simulink model "DSB"  (R2022a)
settings: Solver=VariableStepAuto  StartTime=0.0  StopTime=9  RelTol=1e-3
InitFcn:
  | dsb_init()
StopFcn:
  | dsb_plots()
  | dsb_play()
libraries: commanapbnd3 x2, commchan3 x1
settings Model: Creator=aliel  LastModifiedBy=aliel

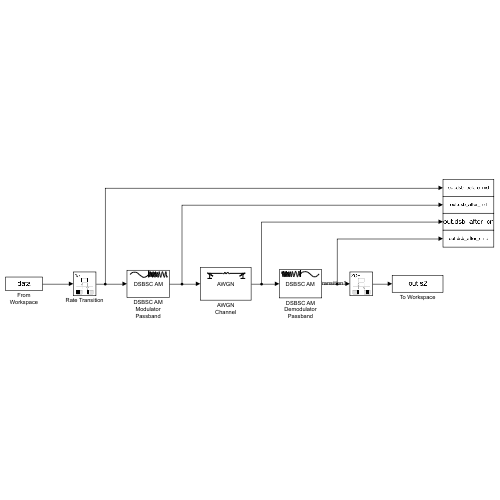
[thumbnail: Simulink's stored preview of the top-level diagram]
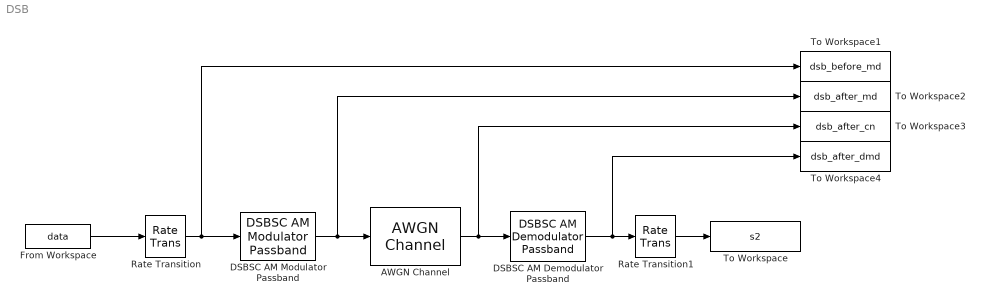
== system DSB ==
  AWGN Channel : commchan3/AWGN Channel  InputProcessing=Columns as channels (frame based)  seed=67  noiseMode="Signal to noise ratio  (SNR)"  EbNodB=10  EsNodB=10  SNRdB=30  bitsPerSym=1  Ps=0.0191  Tsym=1  variance=1
  DSBSC AM Demodulator Passband : commanapbnd3/DSBSC AM Demodulator Passband  Fc=17000  Ph=0  method=Chebyshev I  n=10  cf=4000  Rp=0.1  Rs=50
      settings: SourceProductBaseCode=CM
  DSBSC AM Modulator Passband : commanapbnd3/DSBSC AM Modulator Passband  Fc=17000  Ph=0
      settings: SourceProductBaseCode=CM
  From Workspace : FromWorkspace  VariableName=data  SampleTime=1/8192  OutputAfterFinalValue=Holding final value
  Rate Transition : RateTransition  OutPortSampleTime=1/(10*8192)
  Rate Transition1 : RateTransition  OutPortSampleTime=1/8192
  To Workspace : ToWorkspace  VariableName=s2  SampleTime=-1
      settings: Save2DSignal=2-D array (concatenate along first dimension)
  To Workspace1 : ToWorkspace  VariableName=dsb_before_md  SampleTime=-1
      settings: Save2DSignal=2-D array (concatenate along first dimension)
  To Workspace2 : ToWorkspace  VariableName=dsb_after_md  SampleTime=-1
      settings: Save2DSignal=2-D array (concatenate along first dimension)
  To Workspace3 : ToWorkspace  VariableName=dsb_after_cn  SampleTime=-1
      settings: Save2DSignal=2-D array (concatenate along first dimension)
  To Workspace4 : ToWorkspace  VariableName=dsb_after_dmd  SampleTime=-1
      settings: Save2DSignal=2-D array (concatenate along first dimension)
  wires:
  DSBSC AM Modulator Passband/1 -> To Workspace2/1, AWGN Channel/1
  AWGN Channel/1 -> To Workspace3/1, DSBSC AM Demodulator Passband/1
  From Workspace/1 -> Rate Transition/1
  Rate Transition/1 -> To Workspace1/1, DSBSC AM Modulator Passband/1
  DSBSC AM Demodulator Passband/1 -> To Workspace4/1, Rate Transition1/1
  Rate Transition1/1 -> To Workspace/1
